simulink library "pne_pne3d_generic_std"  (R2016a)
(part 7 of 7)

  pne_pne3d_generic_std_sf/208 -> pne_brk_BrkWearAALt/1  "pne_brk_BrkWearAALt"
  pne_pne3d_generic_std_sf/207 -> pne_brk_Axle4_torque_sns/1  "pne_brk_Axle4_torque_sns"
  pne_pne3d_generic_std_sf/206 -> pne_brk_Axle4_right_Tinterior/1  "pne_brk_Axle4_right_Tinterior"
  pne_pne3d_generic_std_sf/205 -> pne_brk_Axle4_left_Tinterior/1  "pne_brk_Axle4_left_Tinterior"
  pne_pne3d_generic_std_sf/204 -> pne_brk_Axle4_BrakingForce_at8p5bar/1  "pne_brk_Axle4_BrakingForce_at8p5bar"
  pne_pne3d_generic_std_sf/203 -> pne_brk_Axle3_torque_sns/1  "pne_brk_Axle3_torque_sns"
  pne_pne3d_generic_std_sf/202 -> pne_brk_Axle3_right_Tinterior/1  "pne_brk_Axle3_right_Tinterior"
  pne_pne3d_generic_std_sf/201 -> pne_brk_Axle3_left_Tinterior/1  "pne_brk_Axle3_left_Tinterior"
  pne_pne3d_generic_std_sf/200 -> pne_brk_Axle3_BrakingForce_at8p5bar/1  "pne_brk_Axle3_BrakingForce_at8p5bar"
  pne_pne3d_generic_std_sf/199 -> pne_brk_Axle2_torque_sns/1  "pne_brk_Axle2_torque_sns"
  pne_pne3d_generic_std_sf/198 -> pne_brk_Axle2_right_Tinterior/1  "pne_brk_Axle2_right_Tinterior"
  pne_pne3d_generic_std_sf/197 -> pne_brk_Axle2_left_Tinterior/1  "pne_brk_Axle2_left_Tinterior"
  pne_pne3d_generic_std_sf/196 -> pne_brk_Axle2_BrakingForce_at8p5bar/1  "pne_brk_Axle2_BrakingForce_at8p5bar"
  pne_pne3d_generic_std_sf/195 -> pne_brk_Axle1_torque_sns/1  "pne_brk_Axle1_torque_sns"
  pne_pne3d_generic_std_sf/194 -> pne_brk_Axle1_right_Tinterior/1  "pne_brk_Axle1_right_Tinterior"
  pne_pne3d_generic_std_sf/193 -> pne_brk_Axle1_left_Tinterior/1  "pne_brk_Axle1_left_Tinterior"
  pne_pne3d_generic_std_sf/192 -> pne_brk_Axle1_BrakingForce_at8p5bar/1  "pne_brk_Axle1_BrakingForce_at8p5bar"
  pne_pne3d_generic_std_sf/191 -> pne_brk_AdditionalAxle_right_rotVel/1  "pne_brk_AdditionalAxle_right_rotVel"
  pne_pne3d_generic_std_sf/190 -> pne_brk_AdditionalAxle_right_pAct/1  "pne_brk_AdditionalAxle_right_pAct"
  pne_pne3d_generic_std_sf/189 -> pne_brk_AdditionalAxle_left_rotVel/1  "pne_brk_AdditionalAxle_left_rotVel"
  pne_pne3d_generic_std_sf/188 -> pne_brk_AdditionalAxle_left_pAct/1  "pne_brk_AdditionalAxle_left_pAct"
  pne_pne3d_generic_std_sf/187 -> pne_brk_AdditionalAxle_AxMo_right_rotVel/1  "pne_brk_AdditionalAxle_AxMo_right_rotVel"
  pne_pne3d_generic_std_sf/186 -> pne_brk_AdditionalAxle_AxMo_left_rotVel/1  "pne_brk_AdditionalAxle_AxMo_left_rotVel"
  pne_pne3d_generic_std_sf/185 -> pne_brk_Actual_Pressure_TCV/1  "pne_brk_Actual_Pressure_TCV"
  pne_pne3d_generic_std_sf/184 -> pne_brk_Actual_Pressure_RR/1  "pne_brk_Actual_Pressure_RR"
  pne_pne3d_generic_std_sf/183 -> pne_brk_Actual_Pressure_RL/1  "pne_brk_Actual_Pressure_RL"
  pne_pne3d_generic_std_sf/182 -> pne_brk_Actual_Pressure_Rear/1  "pne_brk_Actual_Pressure_Rear"
  pne_pne3d_generic_std_sf/181 -> pne_brk_Actual_Pressure_Front/1  "pne_brk_Actual_Pressure_Front"
  pne_pne3d_generic_std_sf/180 -> pne_brk_Actual_Pressure_FOPB/1  "pne_brk_Actual_Pressure_FOPB"
  pne_pne3d_generic_std_sf/179 -> pne_brk_Actual_Pressure_FA/1  "pne_brk_Actual_Pressure_FA"
  pne_pne3d_generic_std_sf/178 -> pne_brk_Actual_Pressure_AR/1  "pne_brk_Actual_Pressure_AR"
  pne_pne3d_generic_std_sf/177 -> pne_brk_Actual_Pressure_AL/1  "pne_brk_Actual_Pressure_AL"
  pne_pne3d_generic_std_sf/176 -> pne_brk_TrailerAxle3_right_torque/1  "pne_brk_TrailerAxle3_right_torque"
  pne_pne3d_generic_std_sf/175 -> pne_brk_TrailerAxle3_left_torque/1  "pne_brk_TrailerAxle3_left_torque"
  pne_pne3d_generic_std_sf/174 -> pne_brk_TrailerAxle2_right_torque/1  "pne_brk_TrailerAxle2_right_torque"
  pne_pne3d_generic_std_sf/173 -> pne_brk_TrailerAxle2_left_torque/1  "pne_brk_TrailerAxle2_left_torque"
  pne_pne3d_generic_std_sf/172 -> pne_brk_TrailerAxle1_right_torque/1  "pne_brk_TrailerAxle1_right_torque"
  pne_pne3d_generic_std_sf/171 -> pne_brk_TrailerAxle1_left_torque/1  "pne_brk_TrailerAxle1_left_torque"
  pne_pne3d_generic_std_sf/170 -> pne_brk_PowerBoost_Temperature/1  "pne_brk_PowerBoost_Temperature"
  pne_pne3d_generic_std_sf/169 -> pne_brk_PowerBoost_pressure/1  "pne_brk_PowerBoost_pressure"
  pne_pne3d_generic_std_sf/168 -> pne_brk_PowerBoost_massfracH2O/1  "pne_brk_PowerBoost_massfracH2O"
  pne_pne3d_generic_std_sf/167 -> pne_brk_CompressorInlet_mdot/1  "pne_brk_CompressorInlet_mdot"
  pne_pne3d_generic_std_sf/166 -> pne_brk_Axle4_right_torque/1  "pne_brk_Axle4_right_torque"
  pne_pne3d_generic_std_sf/165 -> pne_brk_Axle4_left_torque/1  "pne_brk_Axle4_left_torque"
  pne_pne3d_generic_std_sf/164 -> pne_brk_Axle3_right_torque/1  "pne_brk_Axle3_right_torque"
  pne_pne3d_generic_std_sf/163 -> pne_brk_Axle3_left_torque/1  "pne_brk_Axle3_left_torque"
  pne_pne3d_generic_std_sf/162 -> pne_brk_Axle2_right_torque/1  "pne_brk_Axle2_right_torque"
  pne_pne3d_generic_std_sf/161 -> pne_brk_Axle2_left_torque/1  "pne_brk_Axle2_left_torque"
  pne_pne3d_generic_std_sf/160 -> pne_brk_Axle1_right_torque/1  "pne_brk_Axle1_right_torque"
  pne_pne3d_generic_std_sf/159 -> pne_brk_Axle1_left_torque/1  "pne_brk_Axle1_left_torque"
  pne_pne3d_generic_std_sf/158 -> pne_brk_AirConsumpTx_Temperature/1  "pne_brk_AirConsumpTx_Temperature"
  pne_pne3d_generic_std_sf/157 -> pne_brk_AirConsumpTx_pressure/1  "pne_brk_AirConsumpTx_pressure"
  pne_pne3d_generic_std_sf/156 -> pne_brk_AirConsumpTx_massfracH2O/1  "pne_brk_AirConsumpTx_massfracH2O"
  pne_pne3d_generic_std_sf/155 -> pne_brk_AirConsumpRet_Temperature/1  "pne_brk_AirConsumpRet_Temperature"
  pne_pne3d_generic_std_sf/154 -> pne_brk_AirConsumpRet_pressure/1  "pne_brk_AirConsumpRet_pressure"
  pne_pne3d_generic_std_sf/153 -> pne_brk_AirConsumpRet_massfracH2O/1  "pne_brk_AirConsumpRet_massfracH2O"
  pne_pne3d_generic_std_sf/152 -> pne_brk_AirConsumpEng_Temperature/1  "pne_brk_AirConsumpEng_Temperature"
  pne_pne3d_generic_std_sf/151 -> pne_brk_AirConsumpEng_pressure/1  "pne_brk_AirConsumpEng_pressure"
  pne_pne3d_generic_std_sf/150 -> pne_brk_AirConsumpEng_massfracH2O/1  "pne_brk_AirConsumpEng_massfracH2O"
  pne_pne3d_generic_std_sf/149 -> pne_brk_AirCompressor_torque/1  "pne_brk_AirCompressor_torque"
  pne_pne3d_generic_std_sf/148 -> pne_brk_VTrailer_Temp/1  "pne_brk_VTrailer_Temp"
  pne_pne3d_generic_std_sf/147 -> pne_brk_Vsup_Temp/1  "pne_brk_Vsup_Temp"
  pne_pne3d_generic_std_sf/146 -> pne_brk_Vsup_pRel/1  "pne_brk_Vsup_pRel"
  pne_pne3d_generic_std_sf/145 -> pne_brk_V8_Temp/1  "pne_brk_V8_Temp"
  pne_pne3d_generic_std_sf/144 -> pne_brk_V8_pRel/1  "pne_brk_V8_pRel"
  pne_pne3d_generic_std_sf/143 -> pne_brk_V7_Temp/1  "pne_brk_V7_Temp"
  pne_pne3d_generic_std_sf/142 -> pne_brk_V6_Temp/1  "pne_brk_V6_Temp"
  pne_pne3d_generic_std_sf/141 -> pne_brk_V6_pRel/1  "pne_brk_V6_pRel"
  pne_pne3d_generic_std_sf/140 -> pne_brk_V5_Temp/1  "pne_brk_V5_Temp"
  pne_pne3d_generic_std_sf/139 -> pne_brk_V5_pRel/1  "pne_brk_V5_pRel"
  pne_pne3d_generic_std_sf/138 -> pne_brk_V4_Temp/1  "pne_brk_V4_Temp"
  pne_pne3d_generic_std_sf/137 -> pne_brk_V3_Temp/1  "pne_brk_V3_Temp"
  pne_pne3d_generic_std_sf/136 -> pne_brk_V3_pRel/1  "pne_brk_V3_pRel"
  pne_pne3d_generic_std_sf/135 -> pne_brk_V2_Temp/1  "pne_brk_V2_Temp"
  pne_pne3d_generic_std_sf/134 -> pne_brk_V1_Temp/1  "pne_brk_V1_Temp"
  pne_pne3d_generic_std_sf/133 -> pne_brk_TrailerAxle3Brake_Vol/1  "pne_brk_TrailerAxle3Brake_Vol"
  pne_pne3d_generic_std_sf/132 -> pne_brk_TrailerAxle3Brake_stroke/1  "pne_brk_TrailerAxle3Brake_stroke"
  pne_pne3d_generic_std_sf/131 -> pne_brk_TrailerAxle3Brake_right_pRel/1  "pne_brk_TrailerAxle3Brake_right_pRel"
  pne_pne3d_generic_std_sf/130 -> pne_brk_TrailerAxle3Brake_left_pRel/1  "pne_brk_TrailerAxle3Brake_left_pRel"
  pne_pne3d_generic_std_sf/129 -> pne_brk_TrailerAxle3Brake_Fcyl/1  "pne_brk_TrailerAxle3Brake_Fcyl"
  pne_pne3d_generic_std_sf/128 -> pne_brk_TrailerAxle3_right_torque_grinding/1  "pne_brk_TrailerAxle3_right_torque_grinding"
  pne_pne3d_generic_std_sf/127 -> pne_brk_TrailerAxle3_right_Tinterior/1  "pne_brk_TrailerAxle3_right_Tinterior"
  pne_pne3d_generic_std_sf/126 -> pne_brk_TrailerAxle3_right_Tfriction/1  "pne_brk_TrailerAxle3_right_Tfriction"
  pne_pne3d_generic_std_sf/125 -> pne_brk_TrailerAxle3_right_Tcooldown/1  "pne_brk_TrailerAxle3_right_Tcooldown"
  pne_pne3d_generic_std_sf/124 -> pne_brk_TrailerAxle3_right_sPad_sum/1  "pne_brk_TrailerAxle3_right_sPad_sum"
  pne_pne3d_generic_std_sf/123 -> pne_brk_TrailerAxle3_right_kvT/1  "pne_brk_TrailerAxle3_right_kvT"
  pne_pne3d_generic_std_sf/122 -> pne_brk_TrailerAxle3_left_torque_grinding/1  "pne_brk_TrailerAxle3_left_torque_grinding"
  pne_pne3d_generic_std_sf/121 -> pne_brk_TrailerAxle3_left_Tinterior/1  "pne_brk_TrailerAxle3_left_Tinterior"
  pne_pne3d_generic_std_sf/120 -> pne_brk_TrailerAxle3_left_Tfriction/1  "pne_brk_TrailerAxle3_left_Tfriction"
  pne_pne3d_generic_std_sf/119 -> pne_brk_TrailerAxle3_left_Tcooldown/1  "pne_brk_TrailerAxle3_left_Tcooldown"
  pne_pne3d_generic_std_sf/118 -> pne_brk_TrailerAxle3_left_sPad_sum/1  "pne_brk_TrailerAxle3_left_sPad_sum"
  pne_pne3d_generic_std_sf/117 -> pne_brk_TrailerAxle3_left_kvT/1  "pne_brk_TrailerAxle3_left_kvT"
  pne_pne3d_generic_std_sf/116 -> pne_brk_TrailerAxle3_BrakingPower/1  "pne_brk_TrailerAxle3_BrakingPower"
  pne_pne3d_generic_std_sf/115 -> pne_brk_TrailerAxle2Brake_Vol/1  "pne_brk_TrailerAxle2Brake_Vol"
  pne_pne3d_generic_std_sf/114 -> pne_brk_TrailerAxle2Brake_stroke/1  "pne_brk_TrailerAxle2Brake_stroke"
  pne_pne3d_generic_std_sf/113 -> pne_brk_TrailerAxle2Brake_right_pRel/1  "pne_brk_TrailerAxle2Brake_right_pRel"
  pne_pne3d_generic_std_sf/112 -> pne_brk_TrailerAxle2Brake_left_pRel/1  "pne_brk_TrailerAxle2Brake_left_pRel"
  pne_pne3d_generic_std_sf/111 -> pne_brk_TrailerAxle2Brake_Fcyl/1  "pne_brk_TrailerAxle2Brake_Fcyl"
  pne_pne3d_generic_std_sf/110 -> pne_brk_TrailerAxle2_right_torque_grinding/1  "pne_brk_TrailerAxle2_right_torque_grinding"
  pne_pne3d_generic_std_sf/109 -> pne_brk_TrailerAxle2_right_Tinterior/1  "pne_brk_TrailerAxle2_right_Tinterior"
  pne_pne3d_generic_std_sf/108 -> pne_brk_TrailerAxle2_right_Tfriction/1  "pne_brk_TrailerAxle2_right_Tfriction"
  pne_pne3d_generic_std_sf/107 -> pne_brk_TrailerAxle2_right_Tcooldown/1  "pne_brk_TrailerAxle2_right_Tcooldown"
  pne_pne3d_generic_std_sf/106 -> pne_brk_TrailerAxle2_right_sPad_sum/1  "pne_brk_TrailerAxle2_right_sPad_sum"
  pne_pne3d_generic_std_sf/105 -> pne_brk_TrailerAxle2_right_kvT/1  "pne_brk_TrailerAxle2_right_kvT"
  pne_pne3d_generic_std_sf/104 -> pne_brk_TrailerAxle2_left_torque_grinding/1  "pne_brk_TrailerAxle2_left_torque_grinding"
  pne_pne3d_generic_std_sf/103 -> pne_brk_TrailerAxle2_left_Tinterior/1  "pne_brk_TrailerAxle2_left_Tinterior"
  pne_pne3d_generic_std_sf/102 -> pne_brk_TrailerAxle2_left_Tfriction/1  "pne_brk_TrailerAxle2_left_Tfriction"
  pne_pne3d_generic_std_sf/101 -> pne_brk_TrailerAxle2_left_Tcooldown/1  "pne_brk_TrailerAxle2_left_Tcooldown"
  pne_pne3d_generic_std_sf/100 -> pne_brk_TrailerAxle2_left_sPad_sum/1  "pne_brk_TrailerAxle2_left_sPad_sum"
  pne_pne3d_generic_std_sf/99 -> pne_brk_TrailerAxle2_left_kvT/1  "pne_brk_TrailerAxle2_left_kvT"
  pne_pne3d_generic_std_sf/98 -> pne_brk_TrailerAxle2_BrakingPower/1  "pne_brk_TrailerAxle2_BrakingPower"
  pne_pne3d_generic_std_sf/97 -> pne_brk_TrailerAxle1Brake_Vol/1  "pne_brk_TrailerAxle1Brake_Vol"
  pne_pne3d_generic_std_sf/96 -> pne_brk_TrailerAxle1Brake_stroke/1  "pne_brk_TrailerAxle1Brake_stroke"
  pne_pne3d_generic_std_sf/95 -> pne_brk_TrailerAxle1Brake_right_pRel/1  "pne_brk_TrailerAxle1Brake_right_pRel"
  pne_pne3d_generic_std_sf/94 -> pne_brk_TrailerAxle1Brake_left_pRel/1  "pne_brk_TrailerAxle1Brake_left_pRel"
  pne_pne3d_generic_std_sf/93 -> pne_brk_TrailerAxle1Brake_Fcyl/1  "pne_brk_TrailerAxle1Brake_Fcyl"
  pne_pne3d_generic_std_sf/92 -> pne_brk_TrailerAxle1_right_torque_grinding/1  "pne_brk_TrailerAxle1_right_torque_grinding"
  pne_pne3d_generic_std_sf/91 -> pne_brk_TrailerAxle1_right_Tinterior/1  "pne_brk_TrailerAxle1_right_Tinterior"
  pne_pne3d_generic_std_sf/90 -> pne_brk_TrailerAxle1_right_Tfriction/1  "pne_brk_TrailerAxle1_right_Tfriction"
  pne_pne3d_generic_std_sf/89 -> pne_brk_TrailerAxle1_right_Tcooldown/1  "pne_brk_TrailerAxle1_right_Tcooldown"
  pne_pne3d_generic_std_sf/88 -> pne_brk_TrailerAxle1_right_sPad_sum/1  "pne_brk_TrailerAxle1_right_sPad_sum"
  pne_pne3d_generic_std_sf/87 -> pne_brk_TrailerAxle1_right_kvT/1  "pne_brk_TrailerAxle1_right_kvT"
  pne_pne3d_generic_std_sf/86 -> pne_brk_TrailerAxle1_left_torque_grinding/1  "pne_brk_TrailerAxle1_left_torque_grinding"
  pne_pne3d_generic_std_sf/85 -> pne_brk_TrailerAxle1_left_Tinterior/1  "pne_brk_TrailerAxle1_left_Tinterior"
  pne_pne3d_generic_std_sf/84 -> pne_brk_TrailerAxle1_left_Tfriction/1  "pne_brk_TrailerAxle1_left_Tfriction"
  pne_pne3d_generic_std_sf/83 -> pne_brk_TrailerAxle1_left_Tcooldown/1  "pne_brk_TrailerAxle1_left_Tcooldown"
  pne_pne3d_generic_std_sf/82 -> pne_brk_TrailerAxle1_left_sPad_sum/1  "pne_brk_TrailerAxle1_left_sPad_sum"
  pne_pne3d_generic_std_sf/81 -> pne_brk_TrailerAxle1_left_kvT/1  "pne_brk_TrailerAxle1_left_kvT"
  pne_pne3d_generic_std_sf/80 -> pne_brk_TrailerAxle1_BrakingPower/1  "pne_brk_TrailerAxle1_BrakingPower"
  pne_pne3d_generic_std_sf/79 -> pne_brk_EAPU_Temp/1  "pne_brk_EAPU_Temp"
  pne_pne3d_generic_std_sf/78 -> pne_brk_EAPU_pRel/1  "pne_brk_EAPU_pRel"
  pne_pne3d_generic_std_sf/77 -> pne_brk_CoolingPipe_Temp/1  "pne_brk_CoolingPipe_Temp"
  pne_pne3d_generic_std_sf/76 -> pne_brk_CoolingPipe_pRel/1  "pne_brk_CoolingPipe_pRel"
  pne_pne3d_generic_std_sf/75 -> pne_brk_CompOut_Temp/1  "pne_brk_CompOut_Temp"
  pne_pne3d_generic_std_sf/74 -> pne_brk_Axle4Brake_Vol/1  "pne_brk_Axle4Brake_Vol"
  pne_pne3d_generic_std_sf/73 -> pne_brk_Axle4Brake_stroke/1  "pne_brk_Axle4Brake_stroke"
  pne_pne3d_generic_std_sf/72 -> pne_brk_Axle4Brake_right_pRel/1  "pne_brk_Axle4Brake_right_pRel"
  pne_pne3d_generic_std_sf/71 -> pne_brk_Axle4Brake_left_pRel/1  "pne_brk_Axle4Brake_left_pRel"
  pne_pne3d_generic_std_sf/70 -> pne_brk_Axle4Brake_Fcyl/1  "pne_brk_Axle4Brake_Fcyl"
  pne_pne3d_generic_std_sf/69 -> pne_brk_Axle4_right_torque_grinding/1  "pne_brk_Axle4_right_torque_grinding"
  pne_pne3d_generic_std_sf/68 -> pne_brk_Axle4_right_Tfriction/1  "pne_brk_Axle4_right_Tfriction"
  pne_pne3d_generic_std_sf/67 -> pne_brk_Axle4_right_Tcooldown/1  "pne_brk_Axle4_right_Tcooldown"
  pne_pne3d_generic_std_sf/66 -> pne_brk_Axle4_right_sPad_sum/1  "pne_brk_Axle4_right_sPad_sum"
  pne_pne3d_generic_std_sf/65 -> pne_brk_Axle4_right_kvT/1  "pne_brk_Axle4_right_kvT"
  pne_pne3d_generic_std_sf/64 -> pne_brk_Axle4_left_torque_grinding/1  "pne_brk_Axle4_left_torque_grinding"
  pne_pne3d_generic_std_sf/63 -> pne_brk_Axle4_left_Tfriction/1  "pne_brk_Axle4_left_Tfriction"
  pne_pne3d_generic_std_sf/62 -> pne_brk_Axle4_left_Tcooldown/1  "pne_brk_Axle4_left_Tcooldown"
  pne_pne3d_generic_std_sf/61 -> pne_brk_Axle4_left_sPad_sum/1  "pne_brk_Axle4_left_sPad_sum"
  pne_pne3d_generic_std_sf/60 -> pne_brk_Axle4_left_kvT/1  "pne_brk_Axle4_left_kvT"
  pne_pne3d_generic_std_sf/59 -> pne_brk_Axle4_BrakingPower/1  "pne_brk_Axle4_BrakingPower"
  pne_pne3d_generic_std_sf/58 -> pne_brk_Axle3Brake_Vol/1  "pne_brk_Axle3Brake_Vol"
  pne_pne3d_generic_std_sf/57 -> pne_brk_Axle3Brake_stroke/1  "pne_brk_Axle3Brake_stroke"
  pne_pne3d_generic_std_sf/56 -> pne_brk_Axle3Brake_right_pRel/1  "pne_brk_Axle3Brake_right_pRel"
  pne_pne3d_generic_std_sf/55 -> pne_brk_Axle3Brake_left_pRel/1  "pne_brk_Axle3Brake_left_pRel"
  pne_pne3d_generic_std_sf/54 -> pne_brk_Axle3Brake_Fcyl/1  "pne_brk_Axle3Brake_Fcyl"
  pne_pne3d_generic_std_sf/53 -> pne_brk_Axle3_right_torque_grinding/1  "pne_brk_Axle3_right_torque_grinding"
  pne_pne3d_generic_std_sf/52 -> pne_brk_Axle3_right_Tfriction/1  "pne_brk_Axle3_right_Tfriction"
  pne_pne3d_generic_std_sf/51 -> pne_brk_Axle3_right_Tcooldown/1  "pne_brk_Axle3_right_Tcooldown"
  pne_pne3d_generic_std_sf/50 -> pne_brk_Axle3_right_sPad_sum/1  "pne_brk_Axle3_right_sPad_sum"
  pne_pne3d_generic_std_sf/49 -> pne_brk_Axle3_right_kvT/1  "pne_brk_Axle3_right_kvT"
  pne_pne3d_generic_std_sf/48 -> pne_brk_Axle3_left_torque_grinding/1  "pne_brk_Axle3_left_torque_grinding"
  pne_pne3d_generic_std_sf/47 -> pne_brk_Axle3_left_Tfriction/1  "pne_brk_Axle3_left_Tfriction"
  pne_pne3d_generic_std_sf/46 -> pne_brk_Axle3_left_Tcooldown/1  "pne_brk_Axle3_left_Tcooldown"
  pne_pne3d_generic_std_sf/45 -> pne_brk_Axle3_left_sPad_sum/1  "pne_brk_Axle3_left_sPad_sum"
  pne_pne3d_generic_std_sf/44 -> pne_brk_Axle3_left_kvT/1  "pne_brk_Axle3_left_kvT"
  pne_pne3d_generic_std_sf/43 -> pne_brk_Axle3_BrakingPower/1  "pne_brk_Axle3_BrakingPower"
  pne_pne3d_generic_std_sf/42 -> pne_brk_Axle2Brake_Vol/1  "pne_brk_Axle2Brake_Vol"
  pne_pne3d_generic_std_sf/41 -> pne_brk_Axle2Brake_stroke/1  "pne_brk_Axle2Brake_stroke"
  pne_pne3d_generic_std_sf/40 -> pne_brk_Axle2Brake_right_pRel/1  "pne_brk_Axle2Brake_right_pRel"
  pne_pne3d_generic_std_sf/39 -> pne_brk_Axle2Brake_left_pRel/1  "pne_brk_Axle2Brake_left_pRel"
  pne_pne3d_generic_std_sf/38 -> pne_brk_Axle2Brake_Fcyl/1  "pne_brk_Axle2Brake_Fcyl"
  pne_pne3d_generic_std_sf/37 -> pne_brk_Axle2_right_torque_grinding/1  "pne_brk_Axle2_right_torque_grinding"
  pne_pne3d_generic_std_sf/36 -> pne_brk_Axle2_right_Tfriction/1  "pne_brk_Axle2_right_Tfriction"
  pne_pne3d_generic_std_sf/35 -> pne_brk_Axle2_right_Tcooldown/1  "pne_brk_Axle2_right_Tcooldown"
  pne_pne3d_generic_std_sf/34 -> pne_brk_Axle2_right_sPad_sum/1  "pne_brk_Axle2_right_sPad_sum"
  pne_pne3d_generic_std_sf/33 -> pne_brk_Axle2_right_kvT/1  "pne_brk_Axle2_right_kvT"
  pne_pne3d_generic_std_sf/32 -> pne_brk_Axle2_left_torque_grinding/1  "pne_brk_Axle2_left_torque_grinding"
  pne_pne3d_generic_std_sf/31 -> pne_brk_Axle2_left_Tfriction/1  "pne_brk_Axle2_left_Tfriction"
  pne_pne3d_generic_std_sf/30 -> pne_brk_Axle2_left_Tcooldown/1  "pne_brk_Axle2_left_Tcooldown"
  pne_pne3d_generic_std_sf/29 -> pne_brk_Axle2_left_sPad_sum/1  "pne_brk_Axle2_left_sPad_sum"
  pne_pne3d_generic_std_sf/28 -> pne_brk_Axle2_left_kvT/1  "pne_brk_Axle2_left_kvT"
  pne_pne3d_generic_std_sf/27 -> pne_brk_Axle2_BrakingPower/1  "pne_brk_Axle2_BrakingPower"
  pne_pne3d_generic_std_sf/26 -> pne_brk_Axle1Brake_Vol/1  "pne_brk_Axle1Brake_Vol"
  pne_pne3d_generic_std_sf/25 -> pne_brk_Axle1Brake_stroke/1  "pne_brk_Axle1Brake_stroke"
  pne_pne3d_generic_std_sf/24 -> pne_brk_Axle1Brake_right_pRel/1  "pne_brk_Axle1Brake_right_pRel"
  pne_pne3d_generic_std_sf/23 -> pne_brk_Axle1Brake_left_pRel/1  "pne_brk_Axle1Brake_left_pRel"
  pne_pne3d_generic_std_sf/22 -> pne_brk_Axle1Brake_Fcyl/1  "pne_brk_Axle1Brake_Fcyl"
  pne_pne3d_generic_std_sf/21 -> pne_brk_Axle1_right_torque_grinding/1  "pne_brk_Axle1_right_torque_grinding"
  pne_pne3d_generic_std_sf/20 -> pne_brk_Axle1_right_Tfriction/1  "pne_brk_Axle1_right_Tfriction"
  pne_pne3d_generic_std_sf/19 -> pne_brk_Axle1_right_Tcooldown/1  "pne_brk_Axle1_right_Tcooldown"
  pne_pne3d_generic_std_sf/18 -> pne_brk_Axle1_right_sPad_sum/1  "pne_brk_Axle1_right_sPad_sum"
  pne_pne3d_generic_std_sf/17 -> pne_brk_Axle1_right_kvT/1  "pne_brk_Axle1_right_kvT"
  pne_pne3d_generic_std_sf/16 -> pne_brk_Axle1_left_torque_grinding/1  "pne_brk_Axle1_left_torque_grinding"
  pne_pne3d_generic_std_sf/15 -> pne_brk_Axle1_left_Tfriction/1  "pne_brk_Axle1_left_Tfriction"
  pne_pne3d_generic_std_sf/14 -> pne_brk_Axle1_left_Tcooldown/1  "pne_brk_Axle1_left_Tcooldown"
  pne_pne3d_generic_std_sf/13 -> pne_brk_Axle1_left_sPad_sum/1  "pne_brk_Axle1_left_sPad_sum"
  pne_pne3d_generic_std_sf/12 -> pne_brk_Axle1_left_kvT/1  "pne_brk_Axle1_left_kvT"
  pne_pne3d_generic_std_sf/11 -> pne_brk_Axle1_BrakingPower/1  "pne_brk_Axle1_BrakingPower"
  pne_pne3d_generic_std_sf/10 -> pne_brk_AirCompressor_delivery/1  "pne_brk_AirCompressor_delivery"
  pne_pne3d_generic_std_sf/9 -> pne_AirConsumptionFlow_SCR/1  "pne_AirConsumptionFlow_SCR"
  pne_pne3d_generic_std_sf/8 -> pne_AirConsumptionFlow_PowerBoost/1  "pne_AirConsumptionFlow_PowerBoost"
  pne_pne3d_generic_std_sf/7 -> pne_AirConsumptionFlow_leakage/1  "pne_AirConsumptionFlow_leakage"
  pne_pne3d_generic_std_sf/6 -> pne_AirConsumptionFlow_gearbox/1  "pne_AirConsumptionFlow_gearbox"
  pne_pne3d_generic_std_sf/5 -> pne_AirConsumptionFlow_engine/1  "pne_AirConsumptionFlow_engine"
  pne_pne3d_generic_std_sf/4 -> pne_AirConsumptionFlow_EnduranceBrakes/1  "pne_AirConsumptionFlow_EnduranceBrakes"
  pne_pne3d_generic_std_sf/3 -> pne_AirConsumptionFlow_doors/1  "pne_AirConsumptionFlow_doors"
  pne_pne3d_generic_std_sf/2 -> pne_AirConsumptionFlow_auxiliaries/1  "pne_AirConsumptionFlow_auxiliaries"
  pne_pne3d_generic_std_sf/1 -> pne_AirConsumptionFlow_AirSuspension/1  "pne_AirConsumptionFlow_AirSuspension"
  pne_brk_TrailerAxle3_right_angVel/1 -> pne_pne3d_generic_std_sf/161  "pne_brk_TrailerAxle3_right_angVel"
  pne_brk_TrailerAxle3_right_angPos/1 -> pne_pne3d_generic_std_sf/160  "pne_brk_TrailerAxle3_right_angPos"
  pne_brk_TrailerAxle3_right_angAcc/1 -> pne_pne3d_generic_std_sf/159  "pne_brk_TrailerAxle3_right_angAcc"
  pne_brk_TrailerAxle3_left_angVel/1 -> pne_pne3d_generic_std_sf/158  "pne_brk_TrailerAxle3_left_angVel"
  pne_brk_TrailerAxle3_left_angPos/1 -> pne_pne3d_generic_std_sf/157  "pne_brk_TrailerAxle3_left_angPos"
  pne_brk_TrailerAxle3_left_angAcc/1 -> pne_pne3d_generic_std_sf/156  "pne_brk_TrailerAxle3_left_angAcc"
  pne_brk_TrailerAxle2_right_angVel/1 -> pne_pne3d_generic_std_sf/155  "pne_brk_TrailerAxle2_right_angVel"
  pne_brk_TrailerAxle2_right_angPos/1 -> pne_pne3d_generic_std_sf/154  "pne_brk_TrailerAxle2_right_angPos"
  pne_brk_TrailerAxle2_right_angAcc/1 -> pne_pne3d_generic_std_sf/153  "pne_brk_TrailerAxle2_right_angAcc"
  pne_brk_TrailerAxle2_left_angVel/1 -> pne_pne3d_generic_std_sf/152  "pne_brk_TrailerAxle2_left_angVel"
  pne_brk_TrailerAxle2_left_angPos/1 -> pne_pne3d_generic_std_sf/151  "pne_brk_TrailerAxle2_left_angPos"
  pne_brk_TrailerAxle2_left_angAcc/1 -> pne_pne3d_generic_std_sf/150  "pne_brk_TrailerAxle2_left_angAcc"
  pne_brk_TrailerAxle1_right_angVel/1 -> pne_pne3d_generic_std_sf/149  "pne_brk_TrailerAxle1_right_angVel"
  pne_brk_TrailerAxle1_right_angPos/1 -> pne_pne3d_generic_std_sf/148  "pne_brk_TrailerAxle1_right_angPos"
  pne_brk_TrailerAxle1_right_angAcc/1 -> pne_pne3d_generic_std_sf/147  "pne_brk_TrailerAxle1_right_angAcc"
  pne_brk_TrailerAxle1_left_angVel/1 -> pne_pne3d_generic_std_sf/146  "pne_brk_TrailerAxle1_left_angVel"
  pne_brk_TrailerAxle1_left_angPos/1 -> pne_pne3d_generic_std_sf/145  "pne_brk_TrailerAxle1_left_angPos"
  pne_brk_TrailerAxle1_left_angAcc/1 -> pne_pne3d_generic_std_sf/144  "pne_brk_TrailerAxle1_left_angAcc"
  pne_brk_PowerBoost_mdot/1 -> pne_pne3d_generic_std_sf/143  "pne_brk_PowerBoost_mdot"
  pne_brk_CompressorInlet_Temperature/1 -> pne_pne3d_generic_std_sf/142  "pne_brk_CompressorInlet_Temperature"
  pne_brk_CompressorInlet_pressure/1 -> pne_pne3d_generic_std_sf/141  "pne_brk_CompressorInlet_pressure"
  pne_brk_CompressorInlet_massfracH2O/1 -> pne_pne3d_generic_std_sf/140  "pne_brk_CompressorInlet_massfracH2O"
  pne_brk_Axle4_right_angVel/1 -> pne_pne3d_generic_std_sf/139  "pne_brk_Axle4_right_angVel"
  pne_brk_Axle4_right_angPos/1 -> pne_pne3d_generic_std_sf/138  "pne_brk_Axle4_right_angPos"
  pne_brk_Axle4_right_angAcc/1 -> pne_pne3d_generic_std_sf/137  "pne_brk_Axle4_right_angAcc"
  pne_brk_Axle4_left_angVel/1 -> pne_pne3d_generic_std_sf/136  "pne_brk_Axle4_left_angVel"
  pne_brk_Axle4_left_angPos/1 -> pne_pne3d_generic_std_sf/135  "pne_brk_Axle4_left_angPos"
  pne_brk_Axle4_left_angAcc/1 -> pne_pne3d_generic_std_sf/134  "pne_brk_Axle4_left_angAcc"
  pne_brk_Axle3_right_angVel/1 -> pne_pne3d_generic_std_sf/133  "pne_brk_Axle3_right_angVel"
  pne_brk_Axle3_right_angPos/1 -> pne_pne3d_generic_std_sf/132  "pne_brk_Axle3_right_angPos"
  pne_brk_Axle3_right_angAcc/1 -> pne_pne3d_generic_std_sf/131  "pne_brk_Axle3_right_angAcc"
  pne_brk_Axle3_left_angVel/1 -> pne_pne3d_generic_std_sf/130  "pne_brk_Axle3_left_angVel"
  pne_brk_Axle3_left_angPos/1 -> pne_pne3d_generic_std_sf/129  "pne_brk_Axle3_left_angPos"
  pne_brk_Axle3_left_angAcc/1 -> pne_pne3d_generic_std_sf/128  "pne_brk_Axle3_left_angAcc"
  pne_brk_Axle2_right_angVel/1 -> pne_pne3d_generic_std_sf/127  "pne_brk_Axle2_right_angVel"
  pne_brk_Axle2_right_angPos/1 -> pne_pne3d_generic_std_sf/126  "pne_brk_Axle2_right_angPos"
  pne_brk_Axle2_right_angAcc/1 -> pne_pne3d_generic_std_sf/125  "pne_brk_Axle2_right_angAcc"
  pne_brk_Axle2_left_angVel/1 -> pne_pne3d_generic_std_sf/124  "pne_brk_Axle2_left_angVel"
  pne_brk_Axle2_left_angPos/1 -> pne_pne3d_generic_std_sf/123  "pne_brk_Axle2_left_angPos"
  pne_brk_Axle2_left_angAcc/1 -> pne_pne3d_generic_std_sf/122  "pne_brk_Axle2_left_angAcc"
  pne_brk_Axle1_right_angVel/1 -> pne_pne3d_generic_std_sf/121  "pne_brk_Axle1_right_angVel"
  pne_brk_Axle1_right_angPos/1 -> pne_pne3d_generic_std_sf/120  "pne_brk_Axle1_right_angPos"
  pne_brk_Axle1_right_angAcc/1 -> pne_pne3d_generic_std_sf/119  "pne_brk_Axle1_right_angAcc"
  pne_brk_Axle1_left_angVel/1 -> pne_pne3d_generic_std_sf/118  "pne_brk_Axle1_left_angVel"
  pne_brk_Axle1_left_angPos/1 -> pne_pne3d_generic_std_sf/117  "pne_brk_Axle1_left_angPos"
  pne_brk_Axle1_left_angAcc/1 -> pne_pne3d_generic_std_sf/116  "pne_brk_Axle1_left_angAcc"
  pne_brk_AirConsumpTx_mdot/1 -> pne_pne3d_generic_std_sf/115  "pne_brk_AirConsumpTx_mdot"
  pne_brk_AirConsumpRet_mdot/1 -> pne_pne3d_generic_std_sf/114  "pne_brk_AirConsumpRet_mdot"
  pne_brk_AirConsumpEng_mdot/1 -> pne_pne3d_generic_std_sf/113  "pne_brk_AirConsumpEng_mdot"
  pne_brk_AirCompressor_angVel/1 -> pne_pne3d_generic_std_sf/112  "pne_brk_AirCompressor_angVel"
  pne_brk_AirCompressor_angPos/1 -> pne_pne3d_generic_std_sf/111  "pne_brk_AirCompressor_angPos"
  pne_brk_AirCompressor_angAcc/1 -> pne_pne3d_generic_std_sf/110  "pne_brk_AirCompressor_angAcc"
  env_Temperature/1 -> pne_pne3d_generic_std_sf/109  "env_Temperature"
  env_pressure/1 -> pne_pne3d_generic_std_sf/108  "env_pressure"
  env_air_frontVel/1 -> pne_pne3d_generic_std_sf/107  "env_air_frontVel"
  pneAux_trailerAxle3_right_stABSOutValve/1 -> pne_pne3d_generic_std_sf/106  "pneAux_trailerAxle3_right_stABSOutValve"
  pneAux_trailerAxle3_right_stABSInValve/1 -> pne_pne3d_generic_std_sf/105  "pneAux_trailerAxle3_right_stABSInValve"
  pneAux_trailerAxle3_load/1 -> pne_pne3d_generic_std_sf/104  "pneAux_trailerAxle3_load"
  pneAux_trailerAxle3_left_stABSOutValve/1 -> pne_pne3d_generic_std_sf/103  "pneAux_trailerAxle3_left_stABSOutValve"
  pneAux_trailerAxle3_left_stABSInValve/1 -> pne_pne3d_generic_std_sf/102  "pneAux_trailerAxle3_left_stABSInValve"
  pneAux_trailerAxle2_right_stABSOutValve/1 -> pne_pne3d_generic_std_sf/101  "pneAux_trailerAxle2_right_stABSOutValve"
  pneAux_trailerAxle2_right_stABSInValve/1 -> pne_pne3d_generic_std_sf/100  "pneAux_trailerAxle2_right_stABSInValve"
  pneAux_trailerAxle2_load/1 -> pne_pne3d_generic_std_sf/99  "pneAux_trailerAxle2_load"
  pneAux_trailerAxle2_left_stABSOutValve/1 -> pne_pne3d_generic_std_sf/98  "pneAux_trailerAxle2_left_stABSOutValve"
  pneAux_trailerAxle2_left_stABSInValve/1 -> pne_pne3d_generic_std_sf/97  "pneAux_trailerAxle2_left_stABSInValve"
  pneAux_trailerAxle1_right_stABSOutValve/1 -> pne_pne3d_generic_std_sf/96  "pneAux_trailerAxle1_right_stABSOutValve"
  pneAux_trailerAxle1_right_stABSInValve/1 -> pne_pne3d_generic_std_sf/95  "pneAux_trailerAxle1_right_stABSInValve"
  pneAux_trailerAxle1_load/1 -> pne_pne3d_generic_std_sf/94  "pneAux_trailerAxle1_load"
  pneAux_trailerAxle1_left_stABSOutValve/1 -> pne_pne3d_generic_std_sf/93  "pneAux_trailerAxle1_left_stABSOutValve"
  pneAux_trailerAxle1_left_stABSInValve/1 -> pne_pne3d_generic_std_sf/92  "pneAux_trailerAxle1_left_stABSInValve"
  pneAux_TCV_pDmd_Rear_Right/1 -> pne_pne3d_generic_std_sf/91  "pneAux_TCV_pDmd_Rear_Right"
  pneAux_TCV_pDmd_Rear_Left/1 -> pne_pne3d_generic_std_sf/90  "pneAux_TCV_pDmd_Rear_Left"
  pneAux_TCV_pDmd_Front_Right/1 -> pne_pne3d_generic_std_sf/89  "pneAux_TCV_pDmd_Front_Right"
  pneAux_TCV_pDmd_Front_Left/1 -> pne_pne3d_generic_std_sf/88  "pneAux_TCV_pDmd_Front_Left"
  pneAux_pSollPkBrk/1 -> pne_pne3d_generic_std_sf/87  "pneAux_pSollPkBrk"
  pneAux_pSoll_TCV_p43/1 -> pne_pne3d_generic_std_sf/86  "pneAux_pSoll_TCV_p43"
  pneAux_EAPU_overrun/1 -> pne_pne3d_generic_std_sf/85  "pneAux_EAPU_overrun"
  pneAux_Drs_Rq/1 -> pne_pne3d_generic_std_sf/84  "pneAux_Drs_Rq"
  pneAux_Axle4_load/1 -> pne_pne3d_generic_std_sf/83  "pneAux_Axle4_load"
  pneAux_Axle3_load/1 -> pne_pne3d_generic_std_sf/82  "pneAux_Axle3_load"
  pneAux_Axle2_load/1 -> pne_pne3d_generic_std_sf/81  "pneAux_Axle2_load"
  pneAux_Axle1_load/1 -> pne_pne3d_generic_std_sf/80  "pneAux_Axle1_load"
  pneAux_A3_Ri_Rq/1 -> pne_pne3d_generic_std_sf/79  "pneAux_A3_Ri_Rq"
  pneAux_A3_LoLi_Rq/1 -> pne_pne3d_generic_std_sf/78  "pneAux_A3_LoLi_Rq"
  pneAux_A3_Le_Rq/1 -> pne_pne3d_generic_std_sf/77  "pneAux_A3_Le_Rq"
  pneAux_A2_Ri_Rq/1 -> pne_pne3d_generic_std_sf/76  "pneAux_A2_Ri_Rq"
  pneAux_A2_LoLi_Rq/1 -> pne_pne3d_generic_std_sf/75  "pneAux_A2_LoLi_Rq"
  pneAux_A2_Le_Rq/1 -> pne_pne3d_generic_std_sf/74  "pneAux_A2_Le_Rq"
  pneAux_A1_Ri_Rq/1 -> pne_pne3d_generic_std_sf/73  "pneAux_A1_Ri_Rq"
  pneAux_A1_LoLi_Rq/1 -> pne_pne3d_generic_std_sf/72  "pneAux_A1_LoLi_Rq"
  pneAux_A1_Le_Rq/1 -> pne_pne3d_generic_std_sf/71  "pneAux_A1_Le_Rq"
  Failure_pneumatic_circuit_RA/1 -> pne_pne3d_generic_std_sf/70  "Failure_pneumatic_circuit_RA"
  Failure_pneumatic_circuit_FA/1 -> pne_pne3d_generic_std_sf/69  "Failure_pneumatic_circuit_FA"
  Failure_electric_circuit_RA/1 -> pne_pne3d_generic_std_sf/68  "Failure_electric_circuit_RA"
  Failure_electric_circuit_FA/1 -> pne_pne3d_generic_std_sf/67  "Failure_electric_circuit_FA"
  Failure_electric_circuit_AA/1 -> pne_pne3d_generic_std_sf/66  "Failure_electric_circuit_AA"
  ebs_TCV_pDmd/1 -> pne_pne3d_generic_std_sf/65  "ebs_TCV_pDmd"
  ebs_st3by2_Second/1 -> pne_pne3d_generic_std_sf/64  "ebs_st3by2_Second"
  ebs_st3by2_First/1 -> pne_pne3d_generic_std_sf/63  "ebs_st3by2_First"
  ebs_sil_RAri_vel/1 -> pne_pne3d_generic_std_sf/62  "ebs_sil_RAri_vel"
  ebs_sil_RAri_force/1 -> pne_pne3d_generic_std_sf/61  "ebs_sil_RAri_force"
  ebs_sil_RAle_vel/1 -> pne_pne3d_generic_std_sf/60  "ebs_sil_RAle_vel"
  ebs_sil_RAle_force/1 -> pne_pne3d_generic_std_sf/59  "ebs_sil_RAle_force"
  ebs_sil_FAri_vel/1 -> pne_pne3d_generic_std_sf/58  "ebs_sil_FAri_vel"
  ebs_sil_FAri_force/1 -> pne_pne3d_generic_std_sf/57  "ebs_sil_FAri_force"
  ebs_sil_FAle_vel/1 -> pne_pne3d_generic_std_sf/56  "ebs_sil_FAle_vel"
  ebs_sil_FAle_force/1 -> pne_pne3d_generic_std_sf/55  "ebs_sil_FAle_force"
  ebs_sil_AAri_vel/1 -> pne_pne3d_generic_std_sf/54  "ebs_sil_AAri_vel"
  ebs_sil_AAri_force/1 -> pne_pne3d_generic_std_sf/53  "ebs_sil_AAri_force"
  ebs_sil_AAle_vel/1 -> pne_pne3d_generic_std_sf/52  "ebs_sil_AAle_vel"
  ebs_sil_AAle_force/1 -> pne_pne3d_generic_std_sf/51  "ebs_sil_AAle_force"
  ebs_sBSP_stTCVOutValve/1 -> pne_pne3d_generic_std_sf/50  "ebs_sBSP_stTCVOutValve"
  ebs_sBSP_stTCVInValve/1 -> pne_pne3d_generic_std_sf/49  "ebs_sBSP_stTCVInValve"
  ebs_sBSP_stTCVBuValve/1 -> pne_pne3d_generic_std_sf/48  "ebs_sBSP_stTCVBuValve"
  ebs_sBSP_stRCMaxOutValve_Rear/1 -> pne_pne3d_generic_std_sf/47  "ebs_sBSP_stRCMaxOutValve_Rear"
  ebs_sBSP_stRCMaxOutValve_Front/1 -> pne_pne3d_generic_std_sf/46  "ebs_sBSP_stRCMaxOutValve_Front"
  ebs_sBSP_stRCMaxInValve_Rear/1 -> pne_pne3d_generic_std_sf/45  "ebs_sBSP_stRCMaxInValve_Rear"
  ebs_sBSP_stRCMaxInValve_Front/1 -> pne_pne3d_generic_std_sf/44  "ebs_sBSP_stRCMaxInValve_Front"
  ebs_sBSP_stCMaxOutValve_Rear_Right/1 -> pne_pne3d_generic_std_sf/43  "ebs_sBSP_stCMaxOutValve_Rear_Right"
  ebs_sBSP_stCMaxOutValve_Rear_Left/1 -> pne_pne3d_generic_std_sf/42  "ebs_sBSP_stCMaxOutValve_Rear_Left"
  ebs_sBSP_stCMaxInValve_Rear_Right/1 -> pne_pne3d_generic_std_sf/41  "ebs_sBSP_stCMaxInValve_Rear_Right"
  ebs_sBSP_stCMaxInValve_Rear_Left/1 -> pne_pne3d_generic_std_sf/40  "ebs_sBSP_stCMaxInValve_Rear_Left"
  ebs_sBSP_stCMaxBuValve/1 -> pne_pne3d_generic_std_sf/39  "ebs_sBSP_stCMaxBuValve"
  ebs_sBSP_stAxmoOutValve_Rear_Right/1 -> pne_pne3d_generic_std_sf/38  "ebs_sBSP_stAxmoOutValve_Rear_Right"
  ebs_sBSP_stAxmoOutValve_Rear_Left/1 -> pne_pne3d_generic_std_sf/37  "ebs_sBSP_stAxmoOutValve_Rear_Left"
  ebs_sBSP_stAxmoInValve_Rear_Right/1 -> pne_pne3d_generic_std_sf/36  "ebs_sBSP_stAxmoInValve_Rear_Right"
  ebs_sBSP_stAxmoInValve_Rear_Left/1 -> pne_pne3d_generic_std_sf/35  "ebs_sBSP_stAxmoInValve_Rear_Left"
  ebs_sBSP_stAxmoBuValve/1 -> pne_pne3d_generic_std_sf/34  "ebs_sBSP_stAxmoBuValve"
  ebs_sBSP_stAtcCutOffValve/1 -> pne_pne3d_generic_std_sf/33  "ebs_sBSP_stAtcCutOffValve"
  ebs_sBSP_stAPCVOutValve/1 -> pne_pne3d_generic_std_sf/32  "ebs_sBSP_stAPCVOutValve"
  ebs_sBSP_stAPCVInValve/1 -> pne_pne3d_generic_std_sf/31  "ebs_sBSP_stAPCVInValve"
  ebs_sBSP_stAPCVBuValve/1 -> pne_pne3d_generic_std_sf/30  "ebs_sBSP_stAPCVBuValve"
  ebs_sBSP_stABSOutValve_Rear_Right/1 -> pne_pne3d_generic_std_sf/29  "ebs_sBSP_stABSOutValve_Rear_Right"
  ebs_sBSP_stABSOutValve_Rear_Left/1 -> pne_pne3d_generic_std_sf/28  "ebs_sBSP_stABSOutValve_Rear_Left"
  ebs_sBSP_stABSOutValve_RCMax_Rear/1 -> pne_pne3d_generic_std_sf/27  "ebs_sBSP_stABSOutValve_RCMax_Rear"
  ebs_sBSP_stABSOutValve_RCMax_Front/1 -> pne_pne3d_generic_std_sf/26  "ebs_sBSP_stABSOutValve_RCMax_Front"
  ebs_sBSP_stABSOutValve_Front_Right/1 -> pne_pne3d_generic_std_sf/25  "ebs_sBSP_stABSOutValve_Front_Right"
  ebs_sBSP_stABSOutValve_Front_Left/1 -> pne_pne3d_generic_std_sf/24  "ebs_sBSP_stABSOutValve_Front_Left"
  ebs_sBSP_stABSOutValve_Addl_Right/1 -> pne_pne3d_generic_std_sf/23  "ebs_sBSP_stABSOutValve_Addl_Right"
  ebs_sBSP_stABSOutValve_Addl_Left/1 -> pne_pne3d_generic_std_sf/22  "ebs_sBSP_stABSOutValve_Addl_Left"
  ebs_sBSP_stABSInValve_Rear_Right/1 -> pne_pne3d_generic_std_sf/21  "ebs_sBSP_stABSInValve_Rear_Right"
  ebs_sBSP_stABSInValve_Rear_Left/1 -> pne_pne3d_generic_std_sf/20  "ebs_sBSP_stABSInValve_Rear_Left"
  ebs_sBSP_stABSInValve_RCMax_Rear/1 -> pne_pne3d_generic_std_sf/19  "ebs_sBSP_stABSInValve_RCMax_Rear"
  ebs_sBSP_stABSInValve_RCMax_Front/1 -> pne_pne3d_generic_std_sf/18  "ebs_sBSP_stABSInValve_RCMax_Front"
  ebs_sBSP_stABSInValve_Front_Right/1 -> pne_pne3d_generic_std_sf/17  "ebs_sBSP_stABSInValve_Front_Right"
  ebs_sBSP_stABSInValve_Front_Left/1 -> pne_pne3d_generic_std_sf/16  "ebs_sBSP_stABSInValve_Front_Left"
  ebs_sBSP_stABSInValve_Addl_Right/1 -> pne_pne3d_generic_std_sf/15  "ebs_sBSP_stABSInValve_Addl_Right"
  ebs_sBSP_stABSInValve_Addl_Left/1 -> pne_pne3d_generic_std_sf/14  "ebs_sBSP_stABSInValve_Addl_Left"
  ebs_RearAxle_right_setABS/1 -> pne_pne3d_generic_std_sf/13  "ebs_RearAxle_right_setABS"
  ebs_RearAxle_right_pDmd/1 -> pne_pne3d_generic_std_sf/12  "ebs_RearAxle_right_pDmd"
  ebs_RearAxle_left_setABS/1 -> pne_pne3d_generic_std_sf/11  "ebs_RearAxle_left_setABS"
  ebs_RearAxle_left_pDmd/1 -> pne_pne3d_generic_std_sf/10  "ebs_RearAxle_left_pDmd"
  ebs_FrontAxle_right_setABS/1 -> pne_pne3d_generic_std_sf/9  "ebs_FrontAxle_right_setABS"
  ebs_FrontAxle_right_pDmd/1 -> pne_pne3d_generic_std_sf/8  "ebs_FrontAxle_right_pDmd"
  ebs_FrontAxle_left_setABS/1 -> pne_pne3d_generic_std_sf/7  "ebs_FrontAxle_left_setABS"
  ebs_FrontAxle_left_pDmd/1 -> pne_pne3d_generic_std_sf/6  "ebs_FrontAxle_left_pDmd"
  ebs_ESCsens_y_acceleration/1 -> pne_pne3d_generic_std_sf/5  "ebs_ESCsens_y_acceleration"
  ebs_AdditionalAxle_right_setABS/1 -> pne_pne3d_generic_std_sf/4  "ebs_AdditionalAxle_right_setABS"
  ebs_AdditionalAxle_right_pDmd/1 -> pne_pne3d_generic_std_sf/3  "ebs_AdditionalAxle_right_pDmd"
  ebs_AdditionalAxle_left_setABS/1 -> pne_pne3d_generic_std_sf/2  "ebs_AdditionalAxle_left_setABS"
  ebs_AdditionalAxle_left_pDmd/1 -> pne_pne3d_generic_std_sf/1  "ebs_AdditionalAxle_left_pDmd"
